simulink model "Deadbeat"  (R2016b)
settings: Solver=VariableStepAuto  StartTime=0.0  StopTime=0.5  RelTol=1e-3
libraries: powerlib x58
settings Model: Creator=CNK  LastModifiedBy=CNK

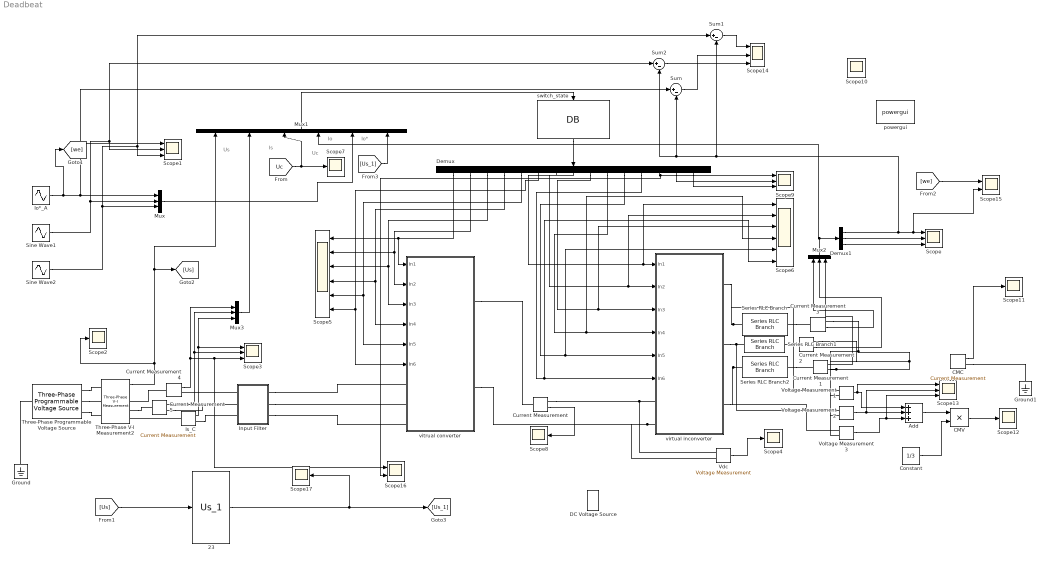
== system Deadbeat ==
  note: Us
  note: Is
  note: Io*
  note: Io
  note: Uc
  "23 " : S-Function  FunctionName=Us_1  SFunctionDeploymentMode=off  EnableBusSupport=off
  Add : Sum  Inputs=3
  CMC : powerlib/Measurements/Current Measurement  PhasorSimulation=off  OutputType=Complex  PSBequivalent=0
  CMV : Product
  Constant : Constant  Value=1/3
  Current Measurement{,1..5} (6 alike) : powerlib/Measurements/Current Measurement  PhasorSimulation=off  OutputType=Complex  PSBequivalent=0
  DC Voltage Source : powerlib/Electrical Sources/DC Voltage Source  Amplitude=120  Measurements=None
  Demux : Demux  Outputs=15
  Demux1 : Demux  Outputs=3
  Ground : powerlib/Elements/Ground  LConnTagsString=a
  Ground1 : powerlib/Elements/Ground  LConnTagsString=a
  Input Filter : Subsystem
  Io*_A : Sin  Amplitude=10  Frequency=10*2*pi  SampleTime=0
  Is_C : powerlib/Measurements/Current Measurement  PhasorSimulation=off  OutputType=Complex  PSBequivalent=0
  Mux : Mux  Inputs=3
  Mux1 : Mux  Inputs=6
  Mux2 : Mux  Inputs=3
  Mux3 : Mux  Inputs=3
  Scope{,1,3,9,13..14} (6 alike) : Scope  NumInputPorts=3
  Scope10 : Scope  NumInputPorts=2
  Scope{2,4,7..8,11..12,17} (7 alike) : Scope
  Scope15 : Scope  NumInputPorts=2
  Scope16 : Scope  NumInputPorts=2
  Scope5 : Scope  NumInputPorts=6
  Scope6 : Scope  NumInputPorts=6
  Series RLC Branch : powerlib/Elements/Series RLC Branch  LConnTagsString=__new0  RConnTagsString=__new0  BranchType=RL  Resistance=2  Inductance=0.02  SetiL0=off  InitialCurrent=0  Capacitance=1e-6  Setx0=off  InitialVoltage=0  Measurements=None
  Series RLC Branch1 : powerlib/Elements/Series RLC Branch  LConnTagsString=__new0  RConnTagsString=__new0  BranchType=RL  Resistance=2  Inductance=0.02  SetiL0=off  InitialCurrent=0  Capacitance=1e-6  Setx0=off  InitialVoltage=0  Measurements=None
  Series RLC Branch2 : powerlib/Elements/Series RLC Branch  LConnTagsString=__new0  RConnTagsString=__new0  BranchType=RL  Resistance=2  Inductance=0.02  SetiL0=off  InitialCurrent=0  Capacitance=1e-6  Setx0=off  InitialVoltage=0  Measurements=None
  Sine Wave1 : Sin  Amplitude=10  Frequency=10*2*pi  Phase=2*pi/3  SampleTime=0
  Sine Wave2 : Sin  Amplitude=10  Frequency=10*2*pi  Phase=4*pi/3  SampleTime=0
  Sum : Sum  Inputs=|+-
  Sum1 : Sum  Inputs=|+-
  Sum2 : Sum  Inputs=|+-
  Three-Phase Programmable Voltage Source : powerlib/Electrical Sources/Three-Phase Programmable Voltage Source  PositiveSequence="[110  0 60]"  VariationEntity=None  VariationType=Table of time-amplitude pairs  VariationTypeAlt=Step  VariationStep=0.5  VariationRate=10  VariationMagnitude=0.3  VariationFrequency=2  VariationTiming=[1 2]  VariationPhaseA=off  Amplitudes=[1 0.8 1.2 1.0]  TimeValues=[0 0.1 0.15 0.2]  HarmonicGeneration=off  HarmonicA=[3 0.2 -25 0]  HarmonicB=[2 0.15 35 2]  Timing="[0.05  3]"  BusType=swing  Pref=0  Qref=0  Qmin=-inf  Qmax=inf
  Three-Phase V-I Measurement2 : powerlib/Measurements/Three-Phase V-I Measurement  VoltageMeasurement=phase-to-ground  SetLabelV=off  LabelV=Vabc  Vpu=off  VpuLL=off  CurrentMeasurement=yes  SetLabelI=off  LabelI=Iabc  Ipu=off  Pbase=100e6  Vbase=500e3  OutputType=Complex  PhasorSimulation=off  PSBequivalent=0
  "Vdc " : powerlib/Measurements/Voltage Measurement  PhasorSimulation=off  OutputType=Complex  PSBequivalent=0
  Voltage Measurement1 : powerlib/Measurements/Voltage Measurement  PhasorSimulation=off  OutputType=Complex  PSBequivalent=0
  Voltage Measurement2 : powerlib/Measurements/Voltage Measurement  PhasorSimulation=off  OutputType=Complex  PSBequivalent=0
  Voltage Measurement3 : powerlib/Measurements/Voltage Measurement  PhasorSimulation=off  OutputType=Complex  PSBequivalent=0
  powergui : powerlib/powergui  Priority=1  SimulationMode=Continuous  SolverType=Tustin/Backward Euler (TBE)  SampleTime=50e-6  frequency=60  SPID=off  DisableSnubberDevices=off  DisableRonSwitches=off  DisableVfSwitches=off  SwTol=0  DisplayEquations=off  Interpol=off  ExternalGateDelay=off  methode=off  Ts=10  FunctionMessages=off  echomessages=off  HookPort=off  EnableUseOfTLC=off  x0status=blocks  frequencyindice=0  Pbase=100e6  ErrMax=1e-4  Iterations=50  UnitsV=kV  UnitsW=MW  buscounter=0  RestoreLinks=warning  ResistiveCurrentMeasurement=off  Frange=[0:2:500]  Ylog=off  Xlog=on  ShowGrid=off  save=off  variable=ZData  structure=Io  ZoomFFT=off  StartTime=0.2  cycles=3  DisplayStyle=1  fundamental=10  FreqAxis=off  MaxFrequency=10000  frequencyindicesteady=1  RmsSteady=1  display=off
  switch_state : S-Function  FunctionName=DB  SFunctionDeploymentMode=off  EnableBusSupport=off
  virtual inconverter : Subsystem
  vitrual converter : Subsystem
  wires:
  Sine Wave1/1 -> Mux/2, Sum2/1, Scope1/2
  Sine Wave2/1 -> Sum1/1, Scope1/3, Mux/3
  Three-Phase V-I Measurement2/1 -> [Us], Mux1/1, Scope2/1
  Mux3/1 -> Mux1/2
  Mux/1 -> Mux1/5
  Mux2/1 -> Mux1/4, Demux1/1
  switch_state/1 -> Demux/1
  Mux1/1 -> switch_state/1
  Demux/1 -> vitrual converter/1(In1), Scope5/1
  Demux/2 -> vitrual converter/2(In2), Scope5/2
  Demux/3 -> vitrual converter/3(In3), Scope5/3
  Demux/4 -> vitrual converter/4(In4), Scope5/4
  Demux/5 -> vitrual converter/5(In5), Scope5/5
  Demux/6 -> vitrual converter/6(In6), Scope5/6
  Demux/7 -> Scope6/1, virtual inconverter/1(In1)
  Demux/9 -> Scope6/3, virtual inconverter/3(In3)
  Demux/10 -> Scope6/4, virtual inconverter/4(In4)
  Demux/11 -> virtual inconverter/5(In5), Scope6/5
  Demux/12 -> virtual inconverter/6(In6), Scope6/6
  Io*_A/1 -> [we], Sum/1, Scope1/1, Mux/1
  "Vdc "/1 -> Scope4/1
  Demux/8 -> Scope6/2, virtual inconverter/2(In2)
  Current Measurement/1 -> Scope8/1
  Demux1/1 -> Sum2/2, Sum/2, Sum1/2, Scope15/2, Scope/1
  Demux1/2 -> Scope/2
  Demux1/3 -> Scope/3
  Sum/1 -> Scope14/2
  Sum1/1 -> Scope14/1
  Sum2/1 -> Scope14/3
  Current Measurement1/1 -> Mux2/3
  Current Measurement3/1 -> Mux2/1
  Current Measurement2/1 -> Mux2/2
  Current Measurement4/1 -> Scope16/1, Scope3/3, Mux3/1
  Current Measurement5/1 -> Scope3/2, Mux3/2
  Is_C/1 -> Scope3/1, Mux3/3
  [Uc] -> Mux1/3, Scope7/1
  CMC/1 -> Scope11/1
  Voltage Measurement1/1 -> Scope13/1, Add/1
  Voltage Measurement2/1 -> Scope13/2, Add/2
  Add/1 -> CMV/1
  Constant/1 -> CMV/2
  CMV/1 -> Scope12/1
  Voltage Measurement3/1 -> Scope13/3, Add/3
  [we] -> Scope15/1
  Demux/13 -> Scope16/2, Scope9/1
  Demux/14 -> Scope9/2
  Demux/15 -> Scope9/3
  [Us] -> "23 "/1
  "23 "/1 -> [Us_1], Scope17/1
  [Us_1] -> Mux1/6
  connections:
  Current Measurement/RConn1 -- "Vdc "/LConn1 -- virtual inconverter/LConn1
  virtual inconverter/LConn2 -- vitrual converter/RConn2 -- "Vdc "/LConn2
  Series RLC Branch/RConn1 -- virtual inconverter/RConn1 -- Voltage Measurement1/LConn1
  Series RLC Branch1/LConn1 -- virtual inconverter/RConn2 -- Voltage Measurement2/LConn1
  Series RLC Branch2/LConn1 -- virtual inconverter/RConn3 -- Voltage Measurement3/LConn1
  Current Measurement3/RConn1 -- Voltage Measurement1/LConn2 -- Voltage Measurement3/LConn2 -- Current Measurement1/RConn1 -- Voltage Measurement2/LConn2 -- Current Measurement2/RConn1
  Series RLC Branch1/RConn1 -- Current Measurement2/LConn1
  Three-Phase Programmable Voltage Source/RConn2 -- Three-Phase V-I Measurement2/LConn2
  Series RLC Branch2/RConn1 -- Current Measurement1/LConn1
  Three-Phase Programmable Voltage Source/LConn1 -- Ground/LConn1
  Three-Phase Programmable Voltage Source/RConn1 -- Three-Phase V-I Measurement2/LConn1
  Input Filter/LConn1 -- Current Measurement4/RConn1
  Series RLC Branch/LConn1 -- Current Measurement3/LConn1
  Is_C/LConn1 -- Three-Phase V-I Measurement2/RConn3
  Three-Phase Programmable Voltage Source/RConn3 -- Three-Phase V-I Measurement2/LConn3
  Current Measurement4/LConn1 -- Three-Phase V-I Measurement2/RConn1
  vitrual converter/RConn1 -- Current Measurement/LConn1
  CMC/RConn1 -- Ground1/LConn1
  Current Measurement5/RConn1 -- Input Filter/LConn2
  Is_C/RConn1 -- Input Filter/LConn3
  Three-Phase V-I Measurement2/RConn2 -- Current Measurement5/LConn1
  Input Filter/RConn1 -- vitrual converter/LConn1
  Input Filter/RConn2 -- vitrual converter/LConn2
  Input Filter/RConn3 -- vitrual converter/LConn3

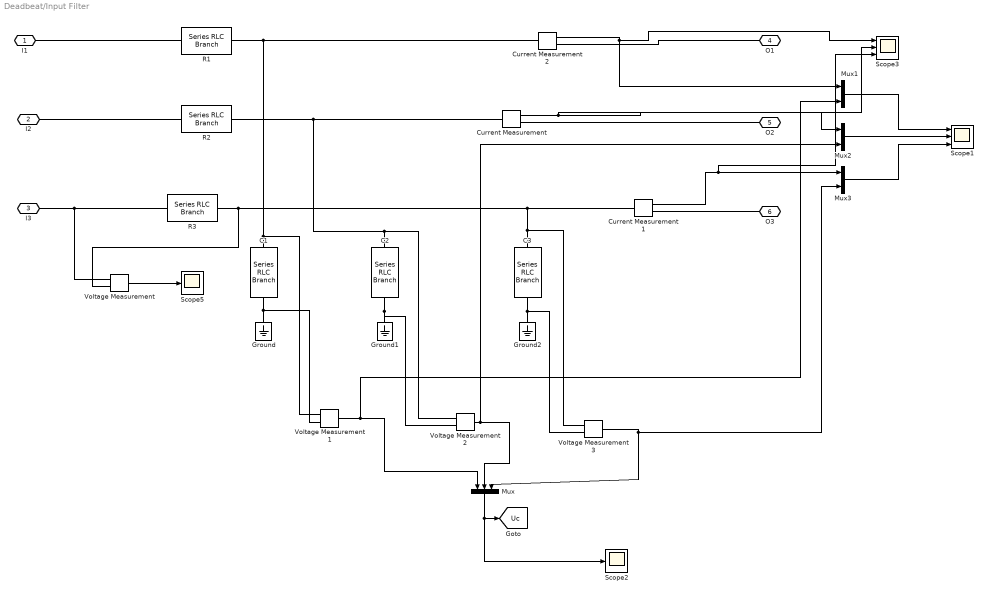
== system Deadbeat/Input Filter ==
  C1 : powerlib/Elements/Series RLC Branch  LConnTagsString=__new0  RConnTagsString=__new0  BranchType=C  Resistance=1  Inductance=1e-3  SetiL0=off  InitialCurrent=0  Capacitance=21e-6  Setx0=off  InitialVoltage=0  Measurements=None
  C2 : powerlib/Elements/Series RLC Branch  LConnTagsString=__new0  RConnTagsString=__new0  BranchType=C  Resistance=1  Inductance=1e-3  SetiL0=off  InitialCurrent=0  Capacitance=21e-6  Setx0=off  InitialVoltage=0  Measurements=None
  C3 : powerlib/Elements/Series RLC Branch  LConnTagsString=__new0  RConnTagsString=__new0  BranchType=C  Resistance=1  Inductance=1e-3  SetiL0=off  InitialCurrent=0  Capacitance=21e-6  Setx0=off  InitialVoltage=0  Measurements=None
  Current Measurement : powerlib/Measurements/Current Measurement  PhasorSimulation=off  OutputType=Complex  PSBequivalent=0
  Current Measurement1 : powerlib/Measurements/Current Measurement  PhasorSimulation=off  OutputType=Complex  PSBequivalent=0
  Current Measurement2 : powerlib/Measurements/Current Measurement  PhasorSimulation=off  OutputType=Complex  PSBequivalent=0
  Ground : powerlib/Elements/Ground  LConnTagsString=a
  Ground1 : powerlib/Elements/Ground  LConnTagsString=a
  Ground2 : powerlib/Elements/Ground  LConnTagsString=a
  Mux : Mux  Inputs=3
  Mux1 : Mux  Inputs=2
  Mux2 : Mux  Inputs=2
  Mux3 : Mux  Inputs=2
  R1 : powerlib/Elements/Series RLC Branch  LConnTagsString=__new0  RConnTagsString=__new0  BranchType=RL  Resistance=2  Inductance=0.0004  SetiL0=off  InitialCurrent=0  Capacitance=5e-6  Setx0=off  InitialVoltage=0  Measurements=None
  R2 : powerlib/Elements/Series RLC Branch  LConnTagsString=__new0  RConnTagsString=__new0  BranchType=RL  Resistance=2  Inductance=0.0004  SetiL0=off  InitialCurrent=0  Capacitance=5e-6  Setx0=off  InitialVoltage=0  Measurements=None
  R3 : powerlib/Elements/Series RLC Branch  LConnTagsString=__new0  RConnTagsString=__new0  BranchType=RL  Resistance=2  Inductance=0.0004  SetiL0=off  InitialCurrent=0  Capacitance=5e-6  Setx0=off  InitialVoltage=0  Measurements=None
  Scope1 : Scope  NumInputPorts=3
  Scope2 : Scope
  Scope3 : Scope  NumInputPorts=3
  Scope5 : Scope
  Voltage Measurement{,1..3} (4 alike) : powerlib/Measurements/Voltage Measurement  PhasorSimulation=off  OutputType=Complex  PSBequivalent=0
  I1 : PMIOPort  Port=1  Side=Left
  I2 : PMIOPort  Port=2  Side=Left
  I3 : PMIOPort  Port=3  Side=Left
  O1 : PMIOPort  Port=4  Side=Right
  O2 : PMIOPort  Port=5  Side=Right
  O3 : PMIOPort  Port=6  Side=Right
  tag scope: Uc=global
  wires:
  Voltage Measurement/1 -> Scope5/1
  Voltage Measurement3/1 -> Mux3/2, Mux/3
  Voltage Measurement2/1 -> Mux2/2, Mux/2
  Voltage Measurement1/1 -> Mux1/2, Mux/1
  Mux/1 -> Scope2/1, [Uc]
  Current Measurement2/1 -> Scope3/1, Mux1/1
  Current Measurement/1 -> Scope3/2, Mux2/1
  Current Measurement1/1 -> Scope3/3, Mux3/1
  Mux2/1 -> Scope1/2
  Mux1/1 -> Scope1/1
  Mux3/1 -> Scope1/3
  connections:
  Voltage Measurement/LConn2 -- Current Measurement1/LConn1 -- Voltage Measurement3/LConn1 -- C3/LConn1 -- R3/RConn1
  C1/LConn1 -- Current Measurement2/LConn1 -- R1/RConn1 -- Voltage Measurement1/LConn1
  R2/RConn1 -- Current Measurement/LConn1 -- C2/LConn1 -- Voltage Measurement2/LConn1
  I2/RConn1 -- R2/LConn1
  I1/RConn1 -- R1/LConn1
  I3/RConn1 -- R3/LConn1 -- Voltage Measurement/LConn1
  Ground/LConn1 -- Voltage Measurement1/LConn2 -- C1/RConn1
  Ground1/LConn1 -- Voltage Measurement2/LConn2 -- C2/RConn1
  Ground2/LConn1 -- Voltage Measurement3/LConn2 -- C3/RConn1
  Current Measurement/RConn1 -- O2/RConn1
  Current Measurement2/RConn1 -- O1/RConn1
  Current Measurement1/RConn1 -- O3/RConn1

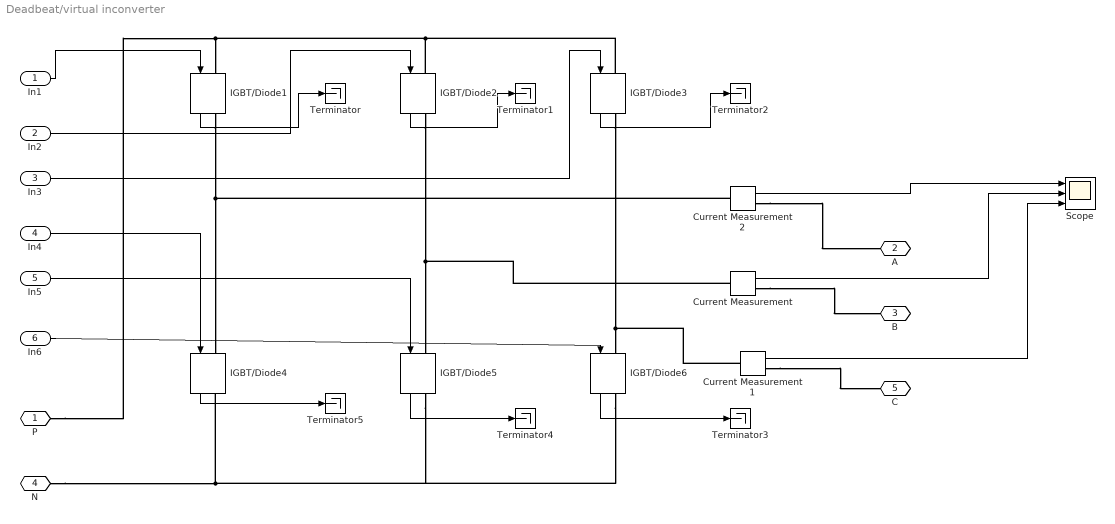
== system Deadbeat/virtual inconverter ==
  In1 : Inport
  In2 : Inport  Port=2
  In3 : Inport  Port=3
  In4 : Inport  Port=4
  In5 : Inport  Port=5
  In6 : Inport  Port=6
  Current Measurement : powerlib/Measurements/Current Measurement  PhasorSimulation=off  OutputType=Complex  PSBequivalent=0
  Current Measurement1 : powerlib/Measurements/Current Measurement  PhasorSimulation=off  OutputType=Complex  PSBequivalent=0
  Current Measurement2 : powerlib/Measurements/Current Measurement  PhasorSimulation=off  OutputType=Complex  PSBequivalent=0
  IGBT/Diode{1..6} (6 alike) : powerlib/Power Electronics/IGBT//Diode  Ron=1e-3  Rs=1e5  Cs=inf  Measurements=on
  Scope : Scope  NumInputPorts=3
  Terminator{,1..5} (6 alike) : Terminator
  P : PMIOPort  Port=1  Side=Left
  A : PMIOPort  Port=2  Side=Right
  B : PMIOPort  Port=3  Side=Right
  N : PMIOPort  Port=4  Side=Left
  C : PMIOPort  Port=5  Side=Right
  wires:
  IGBT/Diode1/1 -> Terminator/1
  IGBT/Diode2/1 -> Terminator1/1
  IGBT/Diode3/1 -> Terminator2/1
  IGBT/Diode6/1 -> Terminator3/1
  IGBT/Diode5/1 -> Terminator4/1
  IGBT/Diode4/1 -> Terminator5/1
  In1/1 -> IGBT/Diode1/1
  In2/1 -> IGBT/Diode2/1
  In3/1 -> IGBT/Diode3/1
  In4/1 -> IGBT/Diode4/1
  In5/1 -> IGBT/Diode5/1
  In6/1 -> IGBT/Diode6/1
  Current Measurement2/1 -> Scope/1
  Current Measurement/1 -> Scope/2
  Current Measurement1/1 -> Scope/3
  connections:
  IGBT/Diode3/LConn1 -- IGBT/Diode2/LConn1 -- P/RConn1 -- IGBT/Diode1/LConn1
  N/RConn1 -- IGBT/Diode6/RConn1 -- IGBT/Diode5/RConn1 -- IGBT/Diode4/RConn1
  IGBT/Diode2/RConn1 -- Current Measurement/LConn1 -- IGBT/Diode5/LConn1
  IGBT/Diode3/RConn1 -- Current Measurement1/LConn1 -- IGBT/Diode6/LConn1
  IGBT/Diode1/RConn1 -- Current Measurement2/LConn1 -- IGBT/Diode4/LConn1
  Current Measurement/RConn1 -- B/RConn1
  Current Measurement1/RConn1 -- C/RConn1
  Current Measurement2/RConn1 -- A/RConn1

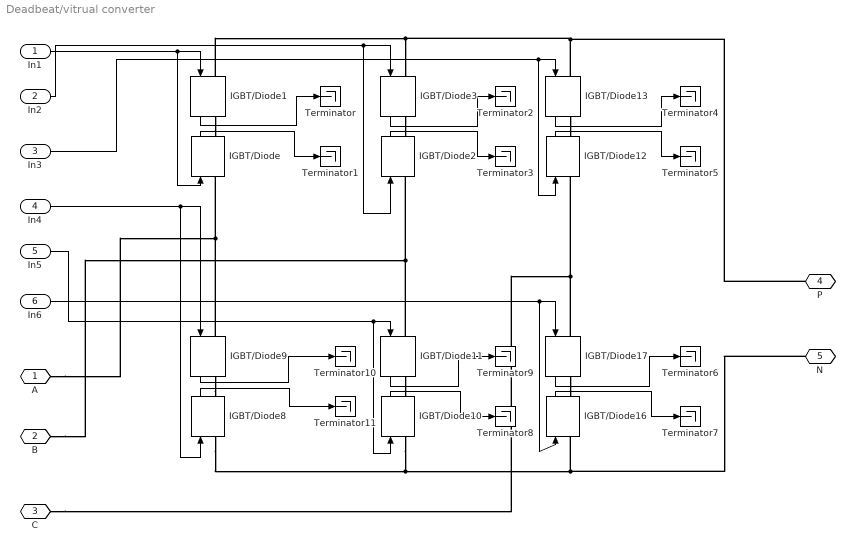
== system Deadbeat/vitrual converter ==
  In1 : Inport
  In2 : Inport  Port=2
  In3 : Inport  Port=3
  In4 : Inport  Port=4
  In5 : Inport  Port=5
  In6 : Inport  Port=6
  IGBT/Diode{,1..3,8..13,16..17} (12 alike) : powerlib/Power Electronics/IGBT//Diode  Ron=1e-3  Rs=1e5  Cs=inf  Measurements=on
  Terminator{,1..11} (12 alike) : Terminator
  A : PMIOPort  Port=1  Side=Left
  B : PMIOPort  Port=2  Side=Left
  C : PMIOPort  Port=3  Side=Left
  P : PMIOPort  Port=4  Side=Right
  N : PMIOPort  Port=5  Side=Right
  wires:
  In1/1 -> IGBT/Diode/1, IGBT/Diode1/1
  IGBT/Diode1/1 -> Terminator/1
  IGBT/Diode/1 -> Terminator1/1
  IGBT/Diode3/1 -> Terminator2/1
  IGBT/Diode2/1 -> Terminator3/1
  IGBT/Diode13/1 -> Terminator4/1
  IGBT/Diode12/1 -> Terminator5/1
  IGBT/Diode17/1 -> Terminator6/1
  IGBT/Diode16/1 -> Terminator7/1
  IGBT/Diode11/1 -> Terminator9/1
  IGBT/Diode10/1 -> Terminator8/1
  IGBT/Diode8/1 -> Terminator11/1
  IGBT/Diode9/1 -> Terminator10/1
  In2/1 -> IGBT/Diode2/1, IGBT/Diode3/1
  In3/1 -> IGBT/Diode12/1, IGBT/Diode13/1
  In4/1 -> IGBT/Diode8/1, IGBT/Diode9/1
  In5/1 -> IGBT/Diode10/1, IGBT/Diode11/1
  In6/1 -> IGBT/Diode16/1, IGBT/Diode17/1
  connections:
  IGBT/Diode1/RConn1 -- IGBT/Diode/RConn1
  IGBT/Diode3/RConn1 -- IGBT/Diode2/RConn1
  IGBT/Diode9/RConn1 -- IGBT/Diode8/RConn1
  IGBT/Diode11/RConn1 -- IGBT/Diode10/RConn1
  IGBT/Diode13/RConn1 -- IGBT/Diode12/RConn1
  IGBT/Diode17/RConn1 -- IGBT/Diode16/RConn1
  IGBT/Diode1/LConn1 -- P/RConn1 -- IGBT/Diode13/LConn1 -- IGBT/Diode3/LConn1
  IGBT/Diode8/LConn1 -- IGBT/Diode16/LConn1 -- N/RConn1 -- IGBT/Diode10/LConn1
  A/RConn1 -- IGBT/Diode9/LConn1 -- IGBT/Diode/LConn1
  IGBT/Diode11/LConn1 -- B/RConn1 -- IGBT/Diode2/LConn1
  IGBT/Diode17/LConn1 -- C/RConn1 -- IGBT/Diode12/LConn1
